simulink model "momentumBasedFlight"  (Simulink 10.3)
settings: Solver=FixedStepAuto  StartTime=0.0  StopTime=Config.simulationTime  FixedStep=Config.tStep  RelTol=1e-3
InitFcn:
  | cd(fileparts(which(bdroot)));
  | initMomentumBasedFlight;
StopFcn:
  | cd(fileparts(which(bdroot)));
  | stopMomentumBasedFlight;
undefined symbols (not defined in the file or in its folder): biasVectorConstraint_feet, Config, confVisualizer, ConstraintMatrix_feet, DiscIntNeverNeededParam, jets_config
undefined symbols (not defined in the file): Frames
libraries: WBToolboxLibrary x25, momentum_flight_control_sublib x2, thrust_estimation_sublib x1, jets_control x1, iDynVisualizer x1
(part 2 of 3)

== system momentumBasedFlight/FLIGHT CONTROLLER (CORE) V2.5 - AERO/Get System State/Change Contact Forces Representation ==
  jointPos : Inport
  w_H_b : Inport  Port=2
  contactForces_WBD : Inport  Port=3
  Change Contact Forces Representation : MATLAB Function  TreatAsAtomicUnit=on
  "CoM6D ->  CoMXYZ1" : Selector  NumberOfDimensions=2  InputPortWidth=7  IndexOptions=Index vector (dialog),Index vector (dialog)  Indices=[1 2 3],[1 2 3]  OutputSizes=1,1
  "CoM6D ->  CoMXYZ3" : Selector  NumberOfDimensions=2  InputPortWidth=7  IndexOptions=Index vector (dialog),Index vector (dialog)  Indices=[1 2 3],[1 2 3]  OutputSizes=1,1
  LFoot Pose : WBToolboxLibrary/Model/Kinematics/ForwardKinematics  frameName=Frames.LFOOT_FRAME
      settings: SourceProductName=WholeBodyToolbox
  Mux : Mux  Inputs=2
  RFoot Pose : WBToolboxLibrary/Model/Kinematics/ForwardKinematics  frameName=Frames.RFOOT_FRAME
      settings: SourceProductName=WholeBodyToolbox
  contactForces : Outport  VectorParamsAs1DForOutWhenUnconnected=off
  tag scope: wrench_LFoot=global, wrench_RFoot=global
  wires:
  contactForces_WBD/1 -> Change Contact Forces Representation/1(contactForces_WBD)
  RFoot Pose/1 -> "CoM6D ->  CoMXYZ3"/1
  "CoM6D ->  CoMXYZ3"/1 -> Change Contact Forces Representation/3(w_R_r_sole)
  LFoot Pose/1 -> "CoM6D ->  CoMXYZ1"/1
  "CoM6D ->  CoMXYZ1"/1 -> Change Contact Forces Representation/2(w_R_l_sole)
  w_H_b/1 -> LFoot Pose/1, RFoot Pose/1
  jointPos/1 -> LFoot Pose/2, RFoot Pose/2
  Change Contact Forces Representation/1(mixed_f_l_sole) -> [wrench_LFoot], Mux/1
  Change Contact Forces Representation/2(mixed_f_r_sole) -> [wrench_RFoot], Mux/2
  Mux/1 -> contactForces/1

== system momentumBasedFlight/Visualizer/Task and Base Frame Kinematics/Combine Rotations ==
  roll : Inport
  pitch : Inport  Port=2
  yaw : Inport  Port=3
  roll_des : Inport  Port=4
  pitch_des : Inport  Port=5
  yaw_des : Inport  Port=6
  Mux : Mux  Inputs=2
  Mux1 : Mux  Inputs=2
  Mux2 : Mux  Inputs=2
  Task rotation combined : Scope  NumInputPorts=3
  wires:
  yaw_des/1 -> Mux2/2
  pitch_des/1 -> Mux1/2
  pitch/1 -> Mux1/1
  roll/1 -> Mux/1
  yaw/1 -> Mux2/1
  roll_des/1 -> Mux/2
  Mux2/1 -> Task rotation combined/3
  Mux1/1 -> Task rotation combined/2
  Mux/1 -> Task rotation combined/1

== system momentumBasedFlight/FLIGHT CONTROLLER (CORE) V2.5 - AERO/Flight Controller RAL-HUMANOIDS V3.0 - AERODYNAMICS/Joint Torque Control for Flying/Integrate Joints Velocity error ==
  jointVel_err : Inport
  Constant : Constant  Value=zeros(Config.N_DOF,1)
  Discrete-Time Integrator1 : DiscreteIntegrator  InitialConditionSource=external  InitialCondition=zeros(Config.N_DOF,1)  SampleTime=Config.tStep  ICPrevOutput=DiscIntNeverNeededParam  ICPrevScaledInput=DiscIntNeverNeededParam
  jointPos_err : Outport  VectorParamsAs1DForOutWhenUnconnected=off
  tag scope: jointPos_err_integral=global
  wires:
  Constant/1 -> Discrete-Time Integrator1/2
  jointVel_err/1 -> Discrete-Time Integrator1/1
  Discrete-Time Integrator1/1 -> [jointPos_err_integral], jointPos_err/1

== system momentumBasedFlight/FLIGHT CONTROLLER (CORE) V2.5 - AERO/Flight Controller RAL-HUMANOIDS V3.0 - AERODYNAMICS/Joint Torque Control for Flying/QP torqueControl ==
  HessianMatrixQP : Inport
  gVectorQP : Inport  Port=2
  ConstraintMatrix_inequality : Inport  Port=3
  biasVectorConstraint_inequality : Inport  Port=4
  feetContactIsActive : Inport  Port=5
  Constant2 : Constant  Value=Config.sat.jointTorquesSaturation
  NOT : Logic  Operator=NOT  IconShape=distinctive  AllPortsSameDT=off  OutDataTypeStr=boolean
  Process QP Inputs Torque Control : MATLAB Function  TreatAsAtomicUnit=on
  QP torqueControl - balancing : Subsystem  TreatAsAtomicUnit=on
  QP torqueControl - flight : Subsystem  TreatAsAtomicUnit=on
  Select QP torqueControl Output : Subsystem
  jointTorques_star : Outport  VectorParamsAs1DForOutWhenUnconnected=off
  exitFlagQP_torqueControl : Outport  Port=2  VectorParamsAs1DForOutWhenUnconnected=off
  wires:
  Select QP torqueControl Output/1(jointTorques_star) -> jointTorques_star/1
  Select QP torqueControl Output/2(exitFlagQP_torqueControl) -> exitFlagQP_torqueControl/1
  QP torqueControl - flight/1(QPStatus_flight) -> Select QP torqueControl Output/4(QPStatus_flight)
  QP torqueControl - flight/2(QPOutput_flight) -> Select QP torqueControl Output/5(QPOutput_flight)
  QP torqueControl - balancing/2(QPOutput_balancing) -> Select QP torqueControl Output/2(QPOutput_balancing)
  QP torqueControl - balancing/1(QPStatus_balancing) -> Select QP torqueControl Output/1(QPStatus_balancing)
  Process QP Inputs Torque Control/1(H_balancing) -> QP torqueControl - balancing/1(H)
  Process QP Inputs Torque Control/2(g_balancing) -> QP torqueControl - balancing/2(g)
  Process QP Inputs Torque Control/3(ub_balancing) -> QP torqueControl - balancing/3(ub)
  Process QP Inputs Torque Control/4(lb_balancing) -> QP torqueControl - balancing/4(lb)
  Process QP Inputs Torque Control/5(Aeq_balancing) -> QP torqueControl - balancing/5(AEq)
  Process QP Inputs Torque Control/6(lbEq_balancing) -> QP torqueControl - balancing/6(lbEq)
  Process QP Inputs Torque Control/7(ubEq_balancing) -> QP torqueControl - balancing/7(ubEq)
  Process QP Inputs Torque Control/11(lb_flight) -> QP torqueControl - flight/4(lb)
  Process QP Inputs Torque Control/10(ub_flight) -> QP torqueControl - flight/3(ub)
  Process QP Inputs Torque Control/9(g_flight) -> QP torqueControl - flight/2(g)
  Process QP Inputs Torque Control/8(H_flight) -> QP torqueControl - flight/1(H)
  Constant2/1 -> Process QP Inputs Torque Control/5(jointTorquesSaturation)
  gVectorQP/1 -> Process QP Inputs Torque Control/2(gVectorQP)
  HessianMatrixQP/1 -> Process QP Inputs Torque Control/1(HessianMatrixQP)
  ConstraintMatrix_inequality/1 -> Process QP Inputs Torque Control/3(InequalityConstrMatrix)
  biasVectorConstraint_inequality/1 -> Process QP Inputs Torque Control/4(biasVectorInequalityConstr)
  NOT/1 -> QP torqueControl - flight/Enable
  feetContactIsActive/1 -> NOT/1, QP torqueControl - balancing/Enable, Select QP torqueControl Output/3(feetContactIsActive)

== system momentumBasedFlight/FLIGHT CONTROLLER (CORE) V2.5 - AERO/Flight Controller RAL-HUMANOIDS V3.0 - AERODYNAMICS/Joint Torque Control for Flying/Torque Derivative Saturation ==
  jointTorques_star : Inport
  Constant1 : Constant  Value=Config.tStep
  Constant2 : Constant  Value=Config.sat.jointTorquesDotMax
  Saturate Torque Derivative : MATLAB Function  TreatAsAtomicUnit=on
  "holder " : WBToolboxLibrary/Utilities/holder 
      settings: SourceProductName=WholeBodyToolbox
  jointTorques_star_sat : Outport  VectorParamsAs1DForOutWhenUnconnected=off
  wires:
  Constant2/1 -> Saturate Torque Derivative/4(uDotMax)
  Constant1/1 -> Saturate Torque Derivative/3(tStep)
  "holder "/1 -> Saturate Torque Derivative/2(u_0)
  Saturate Torque Derivative/1(uSat) -> jointTorques_star_sat/1
  jointTorques_star/1 -> Saturate Torque Derivative/1(u), "holder "/1

== system momentumBasedFlight/FLIGHT CONTROLLER (CORE) V2.5 - AERO/Flight Controller RAL-HUMANOIDS V3.0 - AERODYNAMICS/Momentum Control for Flying/Jet Control ==
  jetDerivatives_des : Inport
  jetsIntensities : Inport  Port=2
  4Jets_EKF : thrust_estimation_sublib/For Test-bench/4Jets_EKF  Config=Config
      settings: SourceProductName=iRonCub Library
  Feedback linearization 4-jets control : jets_control/Feedback linearization 4-jets control  Conf=Config
      settings: SourceProductName=iRonCub Library
  throttle : Outport
  wires:
  4Jets_EKF/1 -> Feedback linearization 4-jets control/1
  Feedback linearization 4-jets control/1 -> throttle/1, 4Jets_EKF/1
  jetsIntensities/1 -> 4Jets_EKF/2
  jetDerivatives_des/1 -> Feedback linearization 4-jets control/2

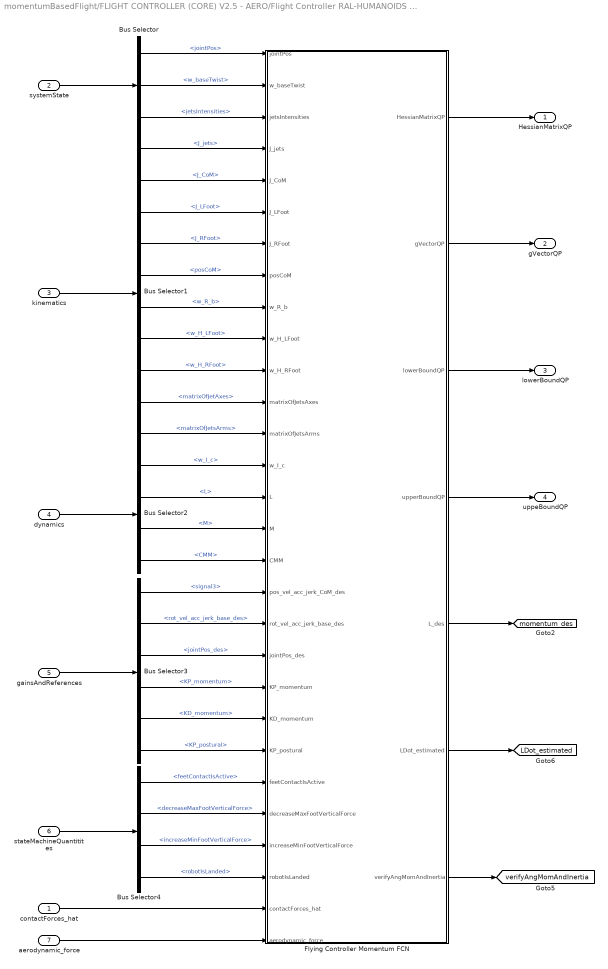
== system momentumBasedFlight/FLIGHT CONTROLLER (CORE) V2.5 - AERO/Flight Controller RAL-HUMANOIDS V3.0 - AERODYNAMICS/Momentum Control for Flying/Momentum Control ==
  contactForces_hat : Inport
  systemState : Inport  Port=2
  kinematics : Inport  Port=3
  dynamics : Inport  Port=4
  gainsAndReferences : Inport  Port=5
  stateMachineQuantitites : Inport  Port=6
  aerodynamic_force : Inport  Port=7
  Bus Selector : BusSelector  OutputSignals=jointPos,w_baseTwist,jetsIntensities
  Bus Selector1 : BusSelector  OutputSignals=J_jets,J_CoM,J_LFoot,J_RFoot,posCoM,w_R_b,w_H_LFoot,w_H_RFoot,matrixOfJetAxes,matrixOfJetsArms
  Bus Selector2 : BusSelector  OutputSignals=w_I_c,L,M,CMM
  Bus Selector3 : BusSelector  OutputSignals=signal3,rot_vel_acc_jerk_base_des,jointPos_des,KP_momentum,KD_momentum,KP_postural
  Bus Selector4 : BusSelector  OutputSignals=feetContactIsActive,decreaseMaxFootVerticalForce,increaseMinFootVerticalForce,robotIsLanded
  "Flying Controller Momentum FCN " : MATLAB Function  TreatAsAtomicUnit=on
  HessianMatrixQP : Outport  VectorParamsAs1DForOutWhenUnconnected=off
  gVectorQP : Outport  Port=2  VectorParamsAs1DForOutWhenUnconnected=off
  lowerBoundQP : Outport  Port=3  VectorParamsAs1DForOutWhenUnconnected=off
  uppeBoundQP : Outport  Port=4  VectorParamsAs1DForOutWhenUnconnected=off
  tag scope: LDot_estimated=global, momentum_des=global, verifyAngMomAndInertia=global
  wires:
  contactForces_hat/1 -> "Flying Controller Momentum FCN "/28(contactForces_hat)
  Bus Selector4/4 -> "Flying Controller Momentum FCN "/27(robotIsLanded)  "<robotIsLanded>"
  Bus Selector4/3 -> "Flying Controller Momentum FCN "/26(increaseMinFootVerticalForce)  "<increaseMinFootVerticalForce>"
  Bus Selector4/2 -> "Flying Controller Momentum FCN "/25(decreaseMaxFootVerticalForce)  "<decreaseMaxFootVerticalForce>"
  Bus Selector2/1 -> "Flying Controller Momentum FCN "/14(w_I_c)  "<w_I_c>"
  Bus Selector1/10 -> "Flying Controller Momentum FCN "/13(matrixOfJetsArms)  "<matrixOfJetsArms>"
  Bus Selector1/9 -> "Flying Controller Momentum FCN "/12(matrixOfJetsAxes)  "<matrixOfJetAxes>"
  Bus Selector3/1 -> "Flying Controller Momentum FCN "/18(pos_vel_acc_jerk_CoM_des)  "<signal3>"
  Bus Selector1/6 -> "Flying Controller Momentum FCN "/9(w_R_b)  "<w_R_b>"
  Bus Selector3/2 -> "Flying Controller Momentum FCN "/19(rot_vel_acc_jerk_base_des)  "<rot_vel_acc_jerk_base_des>"
  Bus Selector1/5 -> "Flying Controller Momentum FCN "/8(posCoM)  "<posCoM>"
  "Flying Controller Momentum FCN "/5(L_des) -> [momentum_des]
  Bus Selector3/6 -> "Flying Controller Momentum FCN "/23(KP_postural)  "<KP_postural>"
  Bus Selector2/2 -> "Flying Controller Momentum FCN "/15(L)  "<L>"
  Bus Selector1/7 -> "Flying Controller Momentum FCN "/10(w_H_LFoot)  "<w_H_LFoot>"
  Bus Selector3/5 -> "Flying Controller Momentum FCN "/22(KD_momentum)  "<KD_momentum>"
  "Flying Controller Momentum FCN "/6(LDot_estimated) -> [LDot_estimated]
  Bus Selector2/3 -> "Flying Controller Momentum FCN "/16(M)  "<M>"
  Bus Selector2/4 -> "Flying Controller Momentum FCN "/17(CMM)  "<CMM>"
  Bus Selector1/8 -> "Flying Controller Momentum FCN "/11(w_H_RFoot)  "<w_H_RFoot>"
  Bus Selector1/4 -> "Flying Controller Momentum FCN "/7(J_RFoot)  "<J_RFoot>"
  Bus Selector/3 -> "Flying Controller Momentum FCN "/3(jetsIntensities)  "<jetsIntensities>"
  gainsAndReferences/1 -> Bus Selector3/1
  Bus Selector1/2 -> "Flying Controller Momentum FCN "/5(J_CoM)  "<J_CoM>"
  dynamics/1 -> Bus Selector2/1
  Bus Selector3/4 -> "Flying Controller Momentum FCN "/21(KP_momentum)  "<KP_momentum>"
  "Flying Controller Momentum FCN "/3(lowerBoundQP) -> lowerBoundQP/1
  stateMachineQuantitites/1 -> Bus Selector4/1
  "Flying Controller Momentum FCN "/7(verifyAngMomAndInertia) -> [verifyAngMomAndInertia]
  Bus Selector4/1 -> "Flying Controller Momentum FCN "/24(feetContactIsActive)  "<feetContactIsActive>"
  "Flying Controller Momentum FCN "/2(gVectorQP) -> gVectorQP/1
  "Flying Controller Momentum FCN "/4(upperBoundQP) -> uppeBoundQP/1
  "Flying Controller Momentum FCN "/1(HessianMatrixQP) -> HessianMatrixQP/1
  Bus Selector/2 -> "Flying Controller Momentum FCN "/2(w_baseTwist)  "<w_baseTwist>"
  Bus Selector1/1 -> "Flying Controller Momentum FCN "/4(J_jets)  "<J_jets>"
  Bus Selector/1 -> "Flying Controller Momentum FCN "/1(jointPos)  "<jointPos>"
  kinematics/1 -> Bus Selector1/1
  Bus Selector1/3 -> "Flying Controller Momentum FCN "/6(J_LFoot)  "<J_LFoot>"
  Bus Selector3/3 -> "Flying Controller Momentum FCN "/20(jointPos_des)  "<jointPos_des>"
  systemState/1 -> Bus Selector/1
  aerodynamic_force/1 -> "Flying Controller Momentum FCN "/29(aerodynamic_force)

== system momentumBasedFlight/FLIGHT CONTROLLER (CORE) V2.5 - AERO/Flight Controller RAL-HUMANOIDS V3.0 - AERODYNAMICS/Momentum Control for Flying/QP Solver and Integrate Contact Forces Derivative ==
  HessianMatrixQP : Inport
  gVectorQP : Inport  Port=2
  lowerBoundQP : Inport  Port=3
  upperBoundQP : Inport  Port=4
  stateMachineQuantities : Inport  Port=5
  systemState : Inport  Port=6
  Bus Selector1 : BusSelector  OutputSignals=feetContactIsActive
  Bus Selector2 : BusSelector  OutputSignals=contactForces
  Integrate the Contact Forces Derivative : Subsystem
  QP momentumControl : Subsystem
  contactForces_star : Outport  VectorParamsAs1DForOutWhenUnconnected=off
  jetsIntensitiesDot_star : Outport  Port=2  VectorParamsAs1DForOutWhenUnconnected=off
  jointVel_star : Outport  Port=3  VectorParamsAs1DForOutWhenUnconnected=off
  tag scope: contactForces_star=global, exitFlagQP_momentumControl=global, jetsIntensitiesDot_star=global, jointVel_star=global
  wires:
  systemState/1 -> Bus Selector2/1
  Bus Selector2/1 -> Integrate the Contact Forces Derivative/2(contactForces)  "<contactForces>"
  Bus Selector1/1 -> Integrate the Contact Forces Derivative/3(feetContactIsActive), QP momentumControl/5(feetContactIsActive)  "<feetContactIsActive>"
  QP momentumControl/3(jointVel_star) -> jointVel_star/1, [jointVel_star]
  QP momentumControl/1(jetsIntensitiesDot_star) -> [jetsIntensitiesDot_star], jetsIntensitiesDot_star/1
  HessianMatrixQP/1 -> QP momentumControl/1(HessianMatrixQP)
  stateMachineQuantities/1 -> Bus Selector1/1
  gVectorQP/1 -> QP momentumControl/2(gVectorQP)
  QP momentumControl/4(exitFlagQP_momentumControl) -> [exitFlagQP_momentumControl]
  upperBoundQP/1 -> QP momentumControl/4(upperBoundQP)
  lowerBoundQP/1 -> QP momentumControl/3(lowerBoundQP)
  QP momentumControl/2(contactForcesDot_star) -> Integrate the Contact Forces Derivative/1(contactForcesDot_star)
  Integrate the Contact Forces Derivative/1(contactForces_star) -> contactForces_star/1, [contactForces_star]

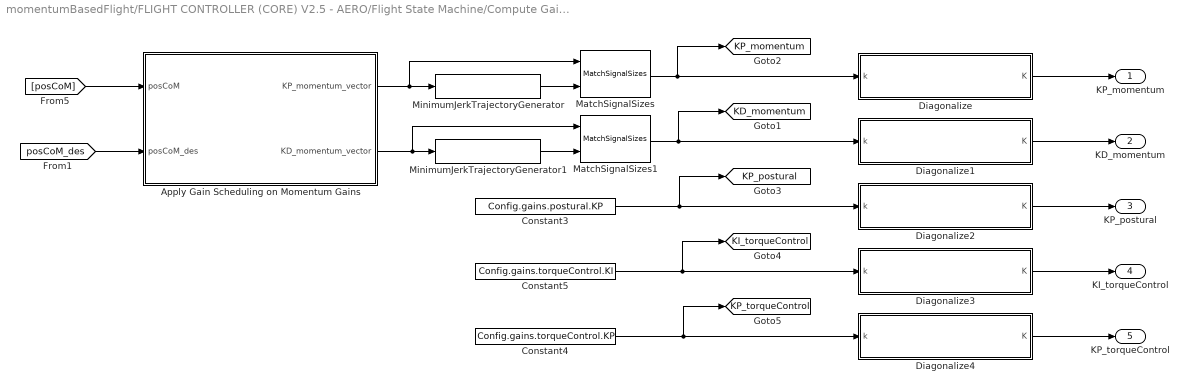
== system momentumBasedFlight/FLIGHT CONTROLLER (CORE) V2.5 - AERO/Flight State Machine/Compute Gains And References/Compute Gains ==
  Apply Gain Scheduling on Momentum Gains : MATLAB Function  TreatAsAtomicUnit=on
  Constant3 : Constant  Value=Config.gains.postural.KP
  Constant4 : Constant  Value=Config.gains.torqueControl.KP
  Constant5 : Constant  Value=Config.gains.torqueControl.KI
  Diagonalize : MATLAB Function  TreatAsAtomicUnit=on
  Diagonalize1 : MATLAB Function  TreatAsAtomicUnit=on
  Diagonalize2 : MATLAB Function  TreatAsAtomicUnit=on
  Diagonalize3 : MATLAB Function  TreatAsAtomicUnit=on
  Diagonalize4 : MATLAB Function  TreatAsAtomicUnit=on
  MatchSignalSizes : WBToolboxLibrary/Utilities/MatchSignalSizes
      settings: SourceProductName=WholeBodyToolbox
  MatchSignalSizes1 : WBToolboxLibrary/Utilities/MatchSignalSizes
      settings: SourceProductName=WholeBodyToolbox
  MinimumJerkTrajectoryGenerator : WBToolboxLibrary/Utilities/MinimumJerkTrajectoryGenerator  externalSettlingTime=off  settlingTime=Config.settlingTime_gainScheduling  sampleTime=Config.tStep  resetOnSettlingTime=off  firstDerivatives=off  secondDerivatives=off  explicitInitialValue=off
      settings: SourceProductName=WholeBodyToolbox
  MinimumJerkTrajectoryGenerator1 : WBToolboxLibrary/Utilities/MinimumJerkTrajectoryGenerator  externalSettlingTime=off  settlingTime=Config.settlingTime_gainScheduling  sampleTime=Config.tStep  resetOnSettlingTime=off  firstDerivatives=off  secondDerivatives=off  explicitInitialValue=off
      settings: SourceProductName=WholeBodyToolbox
  KP_momentum : Outport  VectorParamsAs1DForOutWhenUnconnected=off
  KD_momentum : Outport  Port=2  VectorParamsAs1DForOutWhenUnconnected=off
  KP_postural : Outport  Port=3  VectorParamsAs1DForOutWhenUnconnected=off
  KI_torqueControl : Outport  Port=4  VectorParamsAs1DForOutWhenUnconnected=off
  KP_torqueControl : Outport  Port=5  VectorParamsAs1DForOutWhenUnconnected=off
  tag scope: KD_momentum=global, KI_torqueControl=global, KP_momentum=global, KP_postural=global, KP_torqueControl=global
  wires:
  Constant4/1 -> Diagonalize4/1(k), [KP_torqueControl]
  Constant5/1 -> Diagonalize3/1(k), [KI_torqueControl]
  Constant3/1 -> Diagonalize2/1(k), [KP_postural]
  MatchSignalSizes1/1 -> Diagonalize1/1(k), [KD_momentum]
  MatchSignalSizes/1 -> [KP_momentum], Diagonalize/1(k)
  Diagonalize4/1(K) -> KP_torqueControl/1
  Diagonalize3/1(K) -> KI_torqueControl/1
  Diagonalize2/1(K) -> KP_postural/1
  Diagonalize1/1(K) -> KD_momentum/1
  Diagonalize/1(K) -> KP_momentum/1
  [posCoM] -> Apply Gain Scheduling on Momentum Gains/1(posCoM)
  [posCoM_des] -> Apply Gain Scheduling on Momentum Gains/2(posCoM_des)
  Apply Gain Scheduling on Momentum Gains/1(KP_momentum_vector) -> MatchSignalSizes/1, MinimumJerkTrajectoryGenerator/1
  Apply Gain Scheduling on Momentum Gains/2(KD_momentum_vector) -> MatchSignalSizes1/1, MinimumJerkTrajectoryGenerator1/1
  MinimumJerkTrajectoryGenerator/1 -> MatchSignalSizes/2
  MinimumJerkTrajectoryGenerator1/1 -> MatchSignalSizes1/2

== system momentumBasedFlight/FLIGHT CONTROLLER (CORE) V2.5 - AERO/Flight State Machine/Compute Gains And References/High-speed Flight Trajectory Generator ==
  posCoM_init : Inport
  Clock1 : Clock
  "Trajectory Design for High Speed Motion " : MATLAB Function  TreatAsAtomicUnit=on
  pos_vel_acc_jerk_CoM_des_high_speed : Outport
  turbo_mode_hs : Outport  Port=2
  wires:
  posCoM_init/1 -> "Trajectory Design for High Speed Motion "/2(posCoM_init)
  "Trajectory Design for High Speed Motion "/1(pos_vel_acc_jerk_CoM_des) -> pos_vel_acc_jerk_CoM_des_high_speed/1
  Clock1/1 -> "Trajectory Design for High Speed Motion "/1(t)
  "Trajectory Design for High Speed Motion "/2(turbo_mode_hs) -> turbo_mode_hs/1

== system momentumBasedFlight/FLIGHT CONTROLLER (CORE) V2.5 - AERO/Flight State Machine/Compute Gains And References/Select Planned Trajectory ==
  pos_vel_acc_jerk_CoM_des_ls : Inport
  use_high_speed_traj : Inport  Port=2
  pos_vel_acc_jerk_CoM_des_hs : Inport  Port=3
  Select Trajectory : Switch  Criteria=u2 > Threshold
  pos_vel_acc_jerk_CoM_des : Outport
  wires:
  Select Trajectory/1 -> pos_vel_acc_jerk_CoM_des/1
  use_high_speed_traj/1 -> Select Trajectory/2
  pos_vel_acc_jerk_CoM_des_hs/1 -> Select Trajectory/1
  pos_vel_acc_jerk_CoM_des_ls/1 -> Select Trajectory/3

== system momentumBasedFlight/FLIGHT CONTROLLER (CORE) V2.5 - AERO/Flight State Machine/Compute Gains And References/Smooth CoM and Base References ==
  pos_vel_acc_jerk_CoM_des : Inport
  smoothingTimeCoMPos : Inport  Port=2
  gainSmoothingBaseRot : Inport  Port=3
  rot_vel_acc_jerk_base_des : Inport  Port=4
  Constant : Constant  Value=Config.references.SMOOTH_BASE_ROT_REFERENCES
  Constant1 : Constant  Value=Config.references.SMOOTH_COM_POS_REFERENCES
  Smooth Position References : Subsystem
  Smooth Reference Orientations : Subsystem
  Switch : Switch  Criteria=u2 > Threshold
  Switch2 : Switch  Criteria=u2 > Threshold
  pos_vel_acc_jerk_CoM_des_smooth : Outport  VectorParamsAs1DForOutWhenUnconnected=off
  rot_vel_acc_jerk_base_des_smooth : Outport  Port=2  VectorParamsAs1DForOutWhenUnconnected=off
  wires:
  Constant/1 -> Switch2/2
  Smooth Reference Orientations/1(rot_acc_vel_jerk_base_des_smooth) -> Switch2/1
  gainSmoothingBaseRot/1 -> Smooth Reference Orientations/2(gainSmoothingBaseRot), Switch2/3
  rot_vel_acc_jerk_base_des/1 -> Smooth Reference Orientations/1(rot_vel_acc_jerk_base_des)
  Constant1/1 -> Switch/2
  Switch/1 -> pos_vel_acc_jerk_CoM_des_smooth/1
  Switch2/1 -> rot_vel_acc_jerk_base_des_smooth/1
  pos_vel_acc_jerk_CoM_des/1 -> Smooth Position References/2(pos_vel_acc_jerk_CoM_des), Switch/3
  smoothingTimeCoMPos/1 -> Smooth Position References/1(smoothingTimeCoMPos)
  Smooth Position References/1(pos_vel_acc_jerk_CoM_des_smooth) -> Switch/1

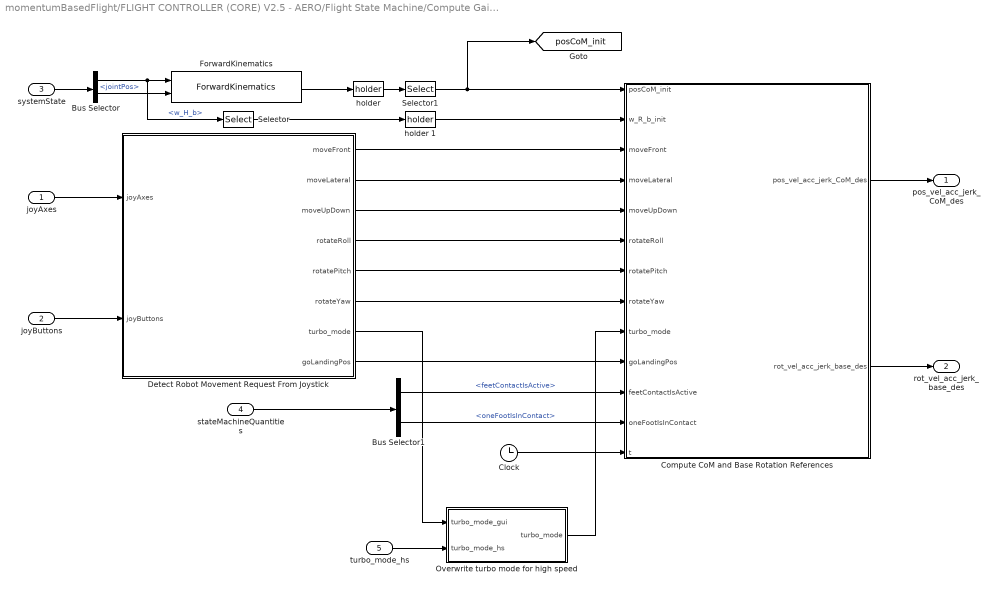
== system momentumBasedFlight/FLIGHT CONTROLLER (CORE) V2.5 - AERO/Flight State Machine/Compute Gains And References/Trajectory Generator ==
  joyAxes : Inport
  joyButtons : Inport  Port=2
  systemState : Inport  Port=3
  stateMachineQuantities : Inport  Port=4
  turbo_mode_hs : Inport  Port=5
  Bus Selector : BusSelector  OutputSignals=w_H_b,jointPos
  Bus Selector1 : BusSelector  OutputSignals=feetContactIsActive,oneFootIsInContact
  Clock : Clock
  Compute CoM and Base Rotation References : MATLAB Function  TreatAsAtomicUnit=on
  Detect Robot Movement Request From Joystick : MATLAB Function  TreatAsAtomicUnit=on
  ForwardKinematics : WBToolboxLibrary/Model/Kinematics/ForwardKinematics  frameName=Frames.COM_FRAME
      settings: SourceProductName=WholeBodyToolbox
  Overwrite turbo mode for high speed : Subsystem
  Selector : Selector  NumberOfDimensions=2  InputPortWidth=3  IndexOptions=Index vector (dialog),Index vector (dialog)  Indices=[1 2 3],[1 2 3]  OutputSizes=1,1
  Selector1 : Selector  NumberOfDimensions=2  InputPortWidth=3  IndexOptions=Index vector (dialog),Index vector (dialog)  Indices=[1 2 3],[4]  OutputSizes=1,1
  "holder " : WBToolboxLibrary/Utilities/holder 
      settings: SourceProductName=WholeBodyToolbox
  holder 1 : WBToolboxLibrary/Utilities/holder 
      settings: SourceProductName=WholeBodyToolbox
  pos_vel_acc_jerk_CoM_des : Outport  VectorParamsAs1DForOutWhenUnconnected=off
  rot_vel_acc_jerk_base_des : Outport  Port=2  VectorParamsAs1DForOutWhenUnconnected=off
  tag scope: posCoM_init=global
  wires:
  Detect Robot Movement Request From Joystick/7(turbo_mode) -> Overwrite turbo mode for high speed/1(turbo_mode_gui)
  Detect Robot Movement Request From Joystick/1(moveFront) -> Compute CoM and Base Rotation References/3(moveFront)
  "holder "/1 -> Selector1/1
  Bus Selector/2 -> ForwardKinematics/2  "<jointPos>"
  Detect Robot Movement Request From Joystick/3(moveUpDown) -> Compute CoM and Base Rotation References/5(moveUpDown)
  Detect Robot Movement Request From Joystick/2(moveLateral) -> Compute CoM and Base Rotation References/4(moveLateral)
  stateMachineQuantities/1 -> Bus Selector1/1
  Detect Robot Movement Request From Joystick/5(rotatePitch) -> Compute CoM and Base Rotation References/7(rotatePitch)
  Bus Selector1/1 -> Compute CoM and Base Rotation References/11(feetContactIsActive)  "<feetContactIsActive>"
  Selector/1 -> holder 1/1
  Bus Selector/1 -> ForwardKinematics/1, Selector/1  "<w_H_b>"
  holder 1/1 -> Compute CoM and Base Rotation References/2(w_R_b_init)
  ForwardKinematics/1 -> "holder "/1
  Detect Robot Movement Request From Joystick/4(rotateRoll) -> Compute CoM and Base Rotation References/6(rotateRoll)
  Compute CoM and Base Rotation References/1(pos_vel_acc_jerk_CoM_des) -> pos_vel_acc_jerk_CoM_des/1
  Detect Robot Movement Request From Joystick/6(rotateYaw) -> Compute CoM and Base Rotation References/8(rotateYaw)
  Clock/1 -> Compute CoM and Base Rotation References/13(t)
  systemState/1 -> Bus Selector/1
  joyAxes/1 -> Detect Robot Movement Request From Joystick/1(joyAxes)
  joyButtons/1 -> Detect Robot Movement Request From Joystick/2(joyButtons)
  Compute CoM and Base Rotation References/2(rot_vel_acc_jerk_base_des) -> rot_vel_acc_jerk_base_des/1
  Selector1/1 -> [posCoM_init], Compute CoM and Base Rotation References/1(posCoM_init)
  Detect Robot Movement Request From Joystick/8(goLandingPos) -> Compute CoM and Base Rotation References/10(goLandingPos)
  Bus Selector1/2 -> Compute CoM and Base Rotation References/12(oneFootIsInContact)  "<oneFootIsInContact>"
  turbo_mode_hs/1 -> Overwrite turbo mode for high speed/2(turbo_mode_hs)
  Overwrite turbo mode for high speed/1(turbo_mode) -> Compute CoM and Base Rotation References/9(turbo_mode)

== system momentumBasedFlight/FLIGHT CONTROLLER (CORE) V2.5 - AERO/Flight Controller RAL-HUMANOIDS V3.0 - AERODYNAMICS/Joint Torque Control for Flying/QP torqueControl/QP torqueControl - balancing ==
  H : Inport
  g : Inport  Port=2
  ub : Inport  Port=3
  lb : Inport  Port=4
  AEq : Inport  Port=5
  lbEq : Inport  Port=6
  ubEq : Inport  Port=7
  Enable : EnablePort
  Combine Bounds and Inequalities : MATLAB Function  TreatAsAtomicUnit=on
  MatchSignalSizes : WBToolboxLibrary/Utilities/MatchSignalSizes
      settings: SourceProductName=WholeBodyToolbox
  QP : WBToolboxLibrary/Utilities/QP  lbA=on  ubA=on  lb=off  ub=off  computeObjVal=off  stopIfFails=off
      settings: SourceProductName=WholeBodyToolbox
  QPStatus_balancing : Outport  VectorParamsAs1DForOutWhenUnconnected=off
  QPOutput_balancing : Outport  Port=2  VectorParamsAs1DForOutWhenUnconnected=off
  wires:
  Combine Bounds and Inequalities/3(ubEq_combined) -> QP/5
  Combine Bounds and Inequalities/2(lbEq_combined) -> QP/4
  Combine Bounds and Inequalities/1(AEq_combined) -> QP/3
  ub/1 -> Combine Bounds and Inequalities/5(ub)
  lb/1 -> Combine Bounds and Inequalities/4(lb)
  ubEq/1 -> Combine Bounds and Inequalities/3(ubEq)
  lbEq/1 -> Combine Bounds and Inequalities/2(lbEq)
  AEq/1 -> Combine Bounds and Inequalities/1(AEq)
  g/1 -> QP/2, MatchSignalSizes/1
  H/1 -> QP/1
  QP/1 -> MatchSignalSizes/2
  MatchSignalSizes/1 -> QPOutput_balancing/1
  QP/2 -> QPStatus_balancing/1

== system momentumBasedFlight/FLIGHT CONTROLLER (CORE) V2.5 - AERO/Flight Controller RAL-HUMANOIDS V3.0 - AERODYNAMICS/Joint Torque Control for Flying/QP torqueControl/QP torqueControl - flight ==
  H : Inport
  g : Inport  Port=2
  ub : Inport  Port=3
  lb : Inport  Port=4
  Enable : EnablePort
  MatchSignalSizes : WBToolboxLibrary/Utilities/MatchSignalSizes
      settings: SourceProductName=WholeBodyToolbox
  QP : WBToolboxLibrary/Utilities/QP  lbA=off  ubA=off  lb=on  ub=on  computeObjVal=off  stopIfFails=off
      settings: SourceProductName=WholeBodyToolbox
  QPStatus_flight : Outport  VectorParamsAs1DForOutWhenUnconnected=off
  QPOutput_flight : Outport  Port=2  VectorParamsAs1DForOutWhenUnconnected=off
  wires:
  ub/1 -> QP/4
  g/1 -> QP/2, MatchSignalSizes/1
  H/1 -> QP/1
  QP/1 -> MatchSignalSizes/2
  MatchSignalSizes/1 -> QPOutput_flight/1
  lb/1 -> QP/3
  QP/2 -> QPStatus_flight/1

== system momentumBasedFlight/FLIGHT CONTROLLER (CORE) V2.5 - AERO/Flight Controller RAL-HUMANOIDS V3.0 - AERODYNAMICS/Joint Torque Control for Flying/QP torqueControl/Select QP torqueControl Output ==
  QPStatus_balancing : Inport
  QPOutput_balancing : Inport  Port=2
  feetContactIsActive : Inport  Port=3
  QPStatus_flight : Inport  Port=4
  QPOutput_flight : Inport  Port=5
  Demux : Demux  Outputs=[12;Config.N_DOF]
  Switch : Switch  Criteria=u2 > Threshold
  Switch1 : Switch  Criteria=u2 > Threshold
  contactForces_QP : Terminator
  jointTorques_star : Outport  VectorParamsAs1DForOutWhenUnconnected=off
  exitFlagQP_torqueControl : Outport  Port=2  VectorParamsAs1DForOutWhenUnconnected=off
  wires:
  Demux/2 -> Switch1/1
  Demux/1 -> contactForces_QP/1
  QPOutput_flight/1 -> Switch1/3
  QPOutput_balancing/1 -> Demux/1
  Switch/1 -> exitFlagQP_torqueControl/1
  QPStatus_flight/1 -> Switch/3
  QPStatus_balancing/1 -> Switch/1
  feetContactIsActive/1 -> Switch/2, Switch1/2
  Switch1/1 -> jointTorques_star/1

== system momentumBasedFlight/FLIGHT CONTROLLER (CORE) V2.5 - AERO/Flight Controller RAL-HUMANOIDS V3.0 - AERODYNAMICS/Momentum Control for Flying/QP Solver and Integrate Contact Forces Derivative/Integrate the Contact Forces Derivative ==
  contactForcesDot_star : Inport
  contactForces : Inport  Port=2
  feetContactIsActive : Inport  Port=3
  Discrete-Time Integrator1 : DiscreteIntegrator  ExternalReset=either  InitialConditionSource=external  InitialCondition=zeros(6,1)  SampleTime=Config.tStep  ICPrevOutput=DiscIntNeverNeededParam  ICPrevScaledInput=DiscIntNeverNeededParam
  Select Integrator Initial Condition : MATLAB Function  TreatAsAtomicUnit=on
  deadZone : Subsystem
  contactForces_star : Outport  VectorParamsAs1DForOutWhenUnconnected=off
  tag scope: contactForcesDot_star=global
  wires:
  Select Integrator Initial Condition/1(contactForces_0) -> Discrete-Time Integrator1/3
  feetContactIsActive/1 -> Discrete-Time Integrator1/2, Select Integrator Initial Condition/1(feetContactIsActive)
  contactForces/1 -> Select Integrator Initial Condition/2(contactForces)
  deadZone/1(u_cut) -> Discrete-Time Integrator1/1
  contactForcesDot_star/1 -> [contactForcesDot_star], deadZone/1(u)
  Discrete-Time Integrator1/1 -> contactForces_star/1

== system momentumBasedFlight/FLIGHT CONTROLLER (CORE) V2.5 - AERO/Flight Controller RAL-HUMANOIDS V3.0 - AERODYNAMICS/Momentum Control for Flying/QP Solver and Integrate Contact Forces Derivative/QP momentumControl ==
  HessianMatrixQP : Inport
  gVectorQP : Inport  Port=2
  lowerBoundQP : Inport  Port=3
  upperBoundQP : Inport  Port=4
  feetContactIsActive : Inport  Port=5
  NOT : Logic  Operator=NOT  IconShape=distinctive  AllPortsSameDT=off  OutDataTypeStr=boolean
  Process QP Inputs Momentum Control : MATLAB Function  TreatAsAtomicUnit=on
  QP momentumControl - balancing : Subsystem  TreatAsAtomicUnit=on
  QP momentumControl - flight : Subsystem  TreatAsAtomicUnit=on
  Select QP momentumControl Output : Subsystem
  jetsIntensitiesDot_star : Outport  VectorParamsAs1DForOutWhenUnconnected=off
  contactForcesDot_star : Outport  Port=2  VectorParamsAs1DForOutWhenUnconnected=off
  jointVel_star : Outport  Port=3  VectorParamsAs1DForOutWhenUnconnected=off
  exitFlagQP_momentumControl : Outport  Port=4  VectorParamsAs1DForOutWhenUnconnected=off
  wires:
  QP momentumControl - flight/2(QPOutput_flight) -> Select QP momentumControl Output/5(QPOutput_flight)
  QP momentumControl - flight/1(QPStatus_flight) -> Select QP momentumControl Output/4(QPStatus_flight)
  QP momentumControl - balancing/2(QPOutput_balancing) -> Select QP momentumControl Output/2(QPOutput_balancing)
  QP momentumControl - balancing/1(QPStatus_balancing) -> Select QP momentumControl Output/1(QPStatus_balancing)
  Select QP momentumControl Output/4(exitFlagQP_momentumControl) -> exitFlagQP_momentumControl/1
  NOT/1 -> QP momentumControl - flight/Enable
  Process QP Inputs Momentum Control/8(lb_flight) -> QP momentumControl - flight/4(lb)
  Process QP Inputs Momentum Control/7(ub_flight) -> QP momentumControl - flight/3(ub)
  Process QP Inputs Momentum Control/4(lb_balancing) -> QP momentumControl - balancing/4(lb)
  Process QP Inputs Momentum Control/3(ub_balancing) -> QP momentumControl - balancing/3(ub)
  Process QP Inputs Momentum Control/6(g_flight) -> QP momentumControl - flight/2(g)
  Process QP Inputs Momentum Control/5(H_flight) -> QP momentumControl - flight/1(H)
  Process QP Inputs Momentum Control/2(g_balancing) -> QP momentumControl - balancing/2(g)
  Process QP Inputs Momentum Control/1(H_balancing) -> QP momentumControl - balancing/1(H)
  Select QP momentumControl Output/2(contactForcesDot_star) -> contactForcesDot_star/1
  Select QP momentumControl Output/3(jointVel_star) -> jointVel_star/1
  Select QP momentumControl Output/1(jetsIntensitiesDot_star) -> jetsIntensitiesDot_star/1
  HessianMatrixQP/1 -> Process QP Inputs Momentum Control/1(HessianMatrixQP)
  upperBoundQP/1 -> Process QP Inputs Momentum Control/4(upperBoundQP)
  feetContactIsActive/1 -> QP momentumControl - balancing/Enable, NOT/1, Select QP momentumControl Output/3(feetContactIsActive)
  lowerBoundQP/1 -> Process QP Inputs Momentum Control/3(lowerBoundQP)
  gVectorQP/1 -> Process QP Inputs Momentum Control/2(gVectorQP)

== system momentumBasedFlight/FLIGHT CONTROLLER (CORE) V2.5 - AERO/Flight State Machine/Compute Gains And References/Smooth CoM and Base References/Smooth Position References ==
  smoothingTimeCoMPos : Inport
  pos_vel_acc_jerk_CoM_des : Inport  Port=2
  "CoM6D ->  CoMXYZ5" : Selector  NumberOfDimensions=2  InputPortWidth=7  IndexOptions=Index vector (dialog),Index vector (dialog)  Indices=[1 2 3],[1]  OutputSizes=1,1
  Compute Smooth Jerk Reference : WBToolboxLibrary/Utilities/MinimumJerkTrajectoryGenerator  externalSettlingTime=off  settlingTime=Config.references.com.tSmoothingCoMAcc  sampleTime=Config.tStep  resetOnSettlingTime=off  firstDerivatives=on  secondDerivatives=off  explicitInitialValue=off
      settings: SourceProductName=WholeBodyToolbox
  Matrix Concatenate : Concatenate  NumInputs=4  Mode=Multidimensional array  ConcatenateDimension=2
  MinimumJerkTrajectoryGenerator : WBToolboxLibrary/Utilities/MinimumJerkTrajectoryGenerator  externalSettlingTime=on  settlingTime=3  sampleTime=Config.tStep  resetOnSettlingTime=off  firstDerivatives=on  secondDerivatives=on  explicitInitialValue=off
      settings: SourceProductName=WholeBodyToolbox
  Terminator : Terminator
  pos_vel_acc_jerk_CoM_des_smooth : Outport  VectorParamsAs1DForOutWhenUnconnected=off
  wires:
  Compute Smooth Jerk Reference/2 -> Matrix Concatenate/4
  Compute Smooth Jerk Reference/1 -> Terminator/1
  MinimumJerkTrajectoryGenerator/3 -> Compute Smooth Jerk Reference/1, Matrix Concatenate/3
  MinimumJerkTrajectoryGenerator/2 -> Matrix Concatenate/2
  "CoM6D ->  CoMXYZ5"/1 -> MinimumJerkTrajectoryGenerator/1
  Matrix Concatenate/1 -> pos_vel_acc_jerk_CoM_des_smooth/1
  MinimumJerkTrajectoryGenerator/1 -> Matrix Concatenate/1
  smoothingTimeCoMPos/1 -> MinimumJerkTrajectoryGenerator/2
  pos_vel_acc_jerk_CoM_des/1 -> "CoM6D ->  CoMXYZ5"/1

== system momentumBasedFlight/FLIGHT CONTROLLER (CORE) V2.5 - AERO/Flight State Machine/Compute Gains And References/Smooth CoM and Base References/Smooth Reference Orientations ==
  rot_vel_acc_jerk_base_des : Inport
  gainSmoothingBaseRot : Inport  Port=2
  Matrix Concatenate6 : Concatenate  NumInputs=4  Mode=Multidimensional array  ConcatenateDimension=2
  MinimumJerkTrajectoryGenerator : WBToolboxLibrary/Utilities/MinimumJerkTrajectoryGenerator  externalSettlingTime=off  settlingTime=Config.references.orientation.tSmoothingAngVel  sampleTime=Config.tStep  resetOnSettlingTime=off  firstDerivatives=on  secondDerivatives=on  explicitInitialValue=off
      settings: SourceProductName=WholeBodyToolbox
  Rotational PID Controller : Subsystem
  Selector : Selector  NumberOfDimensions=2  InputPortWidth=3  IndexOptions=Index vector (dialog),Index vector (dialog)  Indices=[1:3],[1:3]  OutputSizes=1,1
  rot_acc_vel_jerk_base_des_smooth : Outport  VectorParamsAs1DForOutWhenUnconnected=off
  wires:
  MinimumJerkTrajectoryGenerator/3 -> Matrix Concatenate6/4
  gainSmoothingBaseRot/1 -> Rotational PID Controller/2(gainSmoothingBaseRot)
  Selector/1 -> Rotational PID Controller/1(w_R_b_des)
  MinimumJerkTrajectoryGenerator/2 -> Matrix Concatenate6/3
  MinimumJerkTrajectoryGenerator/1 -> Matrix Concatenate6/2
  Rotational PID Controller/2(body_omega_b_des_smooth) -> MinimumJerkTrajectoryGenerator/1
  Rotational PID Controller/1(w_R_b_des_smooth) -> Matrix Concatenate6/1
  Matrix Concatenate6/1 -> rot_acc_vel_jerk_base_des_smooth/1
  rot_vel_acc_jerk_base_des/1 -> Selector/1

== system momentumBasedFlight/FLIGHT CONTROLLER (CORE) V2.5 - AERO/Flight State Machine/Compute Gains And References/Trajectory Generator/Overwrite turbo mode for high speed ==
  turbo_mode_gui : Inport
  turbo_mode_hs : Inport  Port=2
  Constant2 : Constant  Value=Config.high_speed_trajectory
  Switch : Switch  Criteria=u2 > Threshold
  turbo_mode : Outport
  wires:
  Switch/1 -> turbo_mode/1
  turbo_mode_gui/1 -> Switch/3
  turbo_mode_hs/1 -> Switch/1
  Constant2/1 -> Switch/2

== system momentumBasedFlight/FLIGHT CONTROLLER (CORE) V2.5 - AERO/Flight Controller RAL-HUMANOIDS V3.0 - AERODYNAMICS/Momentum Control for Flying/QP Solver and Integrate Contact Forces Derivative/Integrate the Contact Forces Derivative/deadZone ==
  u : Inport
  Constant : Constant  Value=Config.sat.deadZoneThreshold
  Deadzone Function : MATLAB Function  TreatAsAtomicUnit=on
  u_cut : Outport  VectorParamsAs1DForOutWhenUnconnected=off
  wires:
  Constant/1 -> Deadzone Function/2(thr)
  u/1 -> Deadzone Function/1(u)
  Deadzone Function/1(y) -> u_cut/1

== system momentumBasedFlight/FLIGHT CONTROLLER (CORE) V2.5 - AERO/Flight Controller RAL-HUMANOIDS V3.0 - AERODYNAMICS/Momentum Control for Flying/QP Solver and Integrate Contact Forces Derivative/QP momentumControl/QP momentumControl - balancing ==
  H : Inport
  g : Inport  Port=2
  ub : Inport  Port=3
  lb : Inport  Port=4
  Enable : EnablePort
  MatchSignalSizes : WBToolboxLibrary/Utilities/MatchSignalSizes
      settings: SourceProductName=WholeBodyToolbox
  QP : WBToolboxLibrary/Utilities/QP  lbA=off  ubA=off  lb=on  ub=on  computeObjVal=off  stopIfFails=off
      settings: SourceProductName=WholeBodyToolbox
  QPStatus_balancing : Outport  VectorParamsAs1DForOutWhenUnconnected=off
  QPOutput_balancing : Outport  Port=2  VectorParamsAs1DForOutWhenUnconnected=off
  wires:
  ub/1 -> QP/4
  g/1 -> QP/2, MatchSignalSizes/1
  H/1 -> QP/1
  QP/1 -> MatchSignalSizes/2
  MatchSignalSizes/1 -> QPOutput_balancing/1
  lb/1 -> QP/3
  QP/2 -> QPStatus_balancing/1

== system momentumBasedFlight/FLIGHT CONTROLLER (CORE) V2.5 - AERO/Flight Controller RAL-HUMANOIDS V3.0 - AERODYNAMICS/Momentum Control for Flying/QP Solver and Integrate Contact Forces Derivative/QP momentumControl/QP momentumControl - flight ==
  H : Inport
  g : Inport  Port=2
  ub : Inport  Port=3
  lb : Inport  Port=4
  Enable : EnablePort
  MatchSignalSizes : WBToolboxLibrary/Utilities/MatchSignalSizes
      settings: SourceProductName=WholeBodyToolbox
  QP : WBToolboxLibrary/Utilities/QP  lbA=off  ubA=off  lb=on  ub=on  computeObjVal=off  stopIfFails=off
      settings: SourceProductName=WholeBodyToolbox
  QPStatus_flight : Outport  VectorParamsAs1DForOutWhenUnconnected=off
  QPOutput_flight : Outport  Port=2  VectorParamsAs1DForOutWhenUnconnected=off
  wires:
  ub/1 -> QP/4
  g/1 -> QP/2, MatchSignalSizes/1
  H/1 -> QP/1
  QP/1 -> MatchSignalSizes/2
  MatchSignalSizes/1 -> QPOutput_flight/1
  lb/1 -> QP/3
  QP/2 -> QPStatus_flight/1

== system momentumBasedFlight/FLIGHT CONTROLLER (CORE) V2.5 - AERO/Flight Controller RAL-HUMANOIDS V3.0 - AERODYNAMICS/Momentum Control for Flying/QP Solver and Integrate Contact Forces Derivative/QP momentumControl/Select QP momentumControl Output ==
  QPStatus_balancing : Inport
  QPOutput_balancing : Inport  Port=2
  feetContactIsActive : Inport  Port=3
  QPStatus_flight : Inport  Port=4
  QPOutput_flight : Inport  Port=5
  Constant : Constant  Value=zeros(12,1)
  Demux : Demux  Outputs=[4;12;Config.N_DOF]
  Demux1 : Demux  Outputs=[4;Config.N_DOF]
  Switch{,1..3} (4 alike) : Switch  Criteria=u2 > Threshold
  jetsIntensitiesDot_star : Outport  VectorParamsAs1DForOutWhenUnconnected=off
  contactForcesDot_star : Outport  Port=2  VectorParamsAs1DForOutWhenUnconnected=off
  jointVel_star : Outport  Port=3  VectorParamsAs1DForOutWhenUnconnected=off
  exitFlagQP_momentumControl : Outport  Port=4  VectorParamsAs1DForOutWhenUnconnected=off
  wires:
  Demux1/2 -> Switch3/3
  Demux/3 -> Switch3/1
  Constant/1 -> Switch2/3
  Demux/2 -> Switch2/1
  Demux1/1 -> Switch1/3
  Demux/1 -> Switch1/1
  QPOutput_flight/1 -> Demux1/1
  QPOutput_balancing/1 -> Demux/1
  Switch/1 -> exitFlagQP_momentumControl/1
  QPStatus_flight/1 -> Switch/3
  QPStatus_balancing/1 -> Switch/1
  feetContactIsActive/1 -> Switch/2, Switch1/2, Switch2/2, Switch3/2
  Switch3/1 -> jointVel_star/1
  Switch1/1 -> jetsIntensitiesDot_star/1
  Switch2/1 -> contactForcesDot_star/1

== system momentumBasedFlight/FLIGHT CONTROLLER (CORE) V2.5 - AERO/Flight State Machine/Compute Gains And References/Smooth CoM and Base References/Smooth Reference Orientations/Rotational PID Controller ==
  w_R_b_des : Inport
  gainSmoothingBaseRot : Inport  Port=2
  Compute Rotation Matrix Derivative : MATLAB Function  TreatAsAtomicUnit=on
  Discrete-Time Integrator2 : DiscreteIntegrator  InitialConditionSource=external  InitialCondition=zeros(3,1)  SampleTime=Config.tStep  ICPrevOutput=DiscIntNeverNeededParam  ICPrevScaledInput=DiscIntNeverNeededParam
  "holder " : WBToolboxLibrary/Utilities/holder 
      settings: SourceProductName=WholeBodyToolbox
  w_R_b_des_smooth : Outport  VectorParamsAs1DForOutWhenUnconnected=off
  body_omega_b_des_smooth : Outport  Port=2  VectorParamsAs1DForOutWhenUnconnected=off
  wires:
  gainSmoothingBaseRot/1 -> Compute Rotation Matrix Derivative/1(gainSmoothingBaseRot)
  Compute Rotation Matrix Derivative/1(b_omega_b) -> body_omega_b_des_smooth/1
  w_R_b_des/1 -> Compute Rotation Matrix Derivative/2(w_R_b_des), "holder "/1
  Discrete-Time Integrator2/1 -> Compute Rotation Matrix Derivative/3(w_R_b), w_R_b_des_smooth/1
  Compute Rotation Matrix Derivative/2(RDot) -> Discrete-Time Integrator2/1
  "holder "/1 -> Discrete-Time Integrator2/2

== matlab function Visualizer/Task and Base Frame Kinematics/MATLAB Function1 ==
  data: RPY_Corr output double; rollPitchYaw input double
function RPY_Corr = correctYawAngleFCN(rollPitchYaw)

    RPY_Corr = correctYawAngle(rollPitchYaw);

end

== matlab function FLIGHT CONTROLLER (CORE) V2.5 - AERO/Flight State Machine/Compute Gains And References/Compute Gains/Diagonalize ==
  data: k input double; K output double
function K = diagonalMatrixFromVectorFCN(k)

    K = wbc.diagonalMatrixFromVector(k);
end

== matlab function Visualizer/Task and Base Frame Kinematics/MATLAB Function3 ==
  data: RPY_Corr output double; rollPitchYaw input double
function RPY_Corr = correctYawAngleFCN(rollPitchYaw)

    RPY_Corr = correctYawAngle(rollPitchYaw);

end

== matlab function Visualizer/Task and Base Frame Kinematics/Get RPY from rotation matrix  ==
  data: w_R_b input double; rollPitchYaw output double
function rollPitchYaw = rollPitchYawFromRotationFCN(w_R_b)

rollPitchYaw = wbc.rollPitchYawFromRotation(w_R_b);

end

== matlab function FLIGHT CONTROLLER (CORE) V2.5 - AERO/Flight State Machine/Compute Gains And References/Compute Gains/Diagonalize1 ==
  data: k input double; K output double
function K = diagonalMatrixFromVectorFCN(k)

    K = wbc.diagonalMatrixFromVector(k);
end

== matlab function Visualizer/Task and Base Frame Kinematics/Get RPY from rotation matrix ==
  data: w_R_b input double; rollPitchYaw output double
function rollPitchYaw = rollPitchYawFromRotationFCN(w_R_b)

rollPitchYaw = wbc.rollPitchYawFromRotation(w_R_b);

end

== matlab function Visualizer/Task and Base Frame Kinematics/Get RPY error norm ==
  data: rot_err input double; rotErr_norm output double
function rotErr_norm = normFCN(rot_err)

rotErr_norm = norm(rot_err);

end

== matlab function FLIGHT CONTROLLER (CORE) V2.5 - AERO/Flight State Machine/Compute Gains And References/Compute Gains/Diagonalize2 ==
  data: k input double; K output double
function K = diagonalMatrixFromVectorFCN(k)

    K = wbc.diagonalMatrixFromVector(k);
end

== matlab function FLIGHT CONTROLLER (CORE) V2.5 - AERO/Flight Controller RAL-HUMANOIDS V3.0 - AERODYNAMICS/Joint Torque Control for Flying/QP torqueControl/Process QP Inputs Torque Control ==
  data: HessianMatrixQP input double; H_balancing output double; gVectorQP input double; InequalityConstrMatrix input double; biasVectorInequalityConstr input double; g_balancing output double; ub_balancing output double; lb_balancing output double; Aeq_balancing output double; lbEq_balancing output double; ubEq_balancing output double; H_flight output double; g_flight output double; ub_flight output double; lb_flight output double; jointTorquesSaturation input double; Config parameter double
function [H_balancing,g_balancing,ub_balancing,lb_balancing,Aeq_balancing,lbEq_balancing,ubEq_balancing, ...
          H_flight,g_flight,ub_flight,lb_flight] = processQPinputTorqueControlFCN ...
                                                       (HessianMatrixQP,gVectorQP,InequalityConstrMatrix, ...
                                                        biasVectorInequalityConstr,jointTorquesSaturation,Config)   
   
[H_balancing,g_balancing,ub_balancing,lb_balancing,Aeq_balancing,lbEq_balancing,ubEq_balancing, ...
          H_flight,g_flight,ub_flight,lb_flight] = iRonCubLib.processQPinputTorqueControl ...
                                                       (HessianMatrixQP,gVectorQP,InequalityConstrMatrix, ...
                                                        biasVectorInequalityConstr,jointTorquesSaturation,Config);     
end

== matlab function Visualizer/Task and Base Frame Kinematics/MATLAB Function2 ==
  data: RPY_Corr output double; rollPitchYaw input double
function RPY_Corr = correctYawAngleFCN(rollPitchYaw)

    RPY_Corr = correctYawAngle(rollPitchYaw);

end

== matlab function FLIGHT CONTROLLER (CORE) V2.5 - AERO/Flight State Machine/Compute Gains And References/Compute Gains/Diagonalize3 ==
  data: k input double; K output double
function K = diagonalMatrixFromVectorFCN(k)

    K = wbc.diagonalMatrixFromVector(k);
end

== matlab function FLIGHT CONTROLLER (CORE) V2.5 - AERO/Flight State Machine/Compute Gains And References/Compute Gains/Diagonalize4 ==
  data: k input double; K output double
function K = diagonalMatrixFromVectorFCN(k)

    K = wbc.diagonalMatrixFromVector(k);
end

== matlab function FLIGHT CONTROLLER (CORE) V2.5 - AERO/Flight State Machine/Compute Gains And References/Trajectory Generator/Compute CoM and Base Rotation References ==
  data: posCoM_init input double; w_R_b_init input double; moveFront input double; pos_vel_acc_jerk_CoM_des output double; moveLateral input double; moveUpDown input double; rotateRoll input double; rotatePitch input double; rotateYaw input double; turbo_mode input double; goLandingPos input double; feetContactIsActive input double; oneFootIsInContact input double; t input double; Config parameter double; rot_vel_acc_jerk_base_des output double
function [pos_vel_acc_jerk_CoM_des, rot_vel_acc_jerk_base_des] = ...
             computeReferencesBaseAndCoMFCN(posCoM_init, w_R_b_init, moveFront, moveLateral, moveUpDown, rotateRoll, rotatePitch, ...
                                            rotateYaw, turbo_mode, goLandingPos, feetContactIsActive, oneFootIsInContact, t, Config)
                                     
    [pos_vel_acc_jerk_CoM_des, rot_vel_acc_jerk_base_des] = ...
        iRonCubLib.computeReferencesBaseAndCoM(posCoM_init, w_R_b_init, moveFront, moveLateral, moveUpDown, rotateRoll, rotatePitch, ...
                                               rotateYaw, turbo_mode, goLandingPos, feetContactIsActive, oneFootIsInContact, t, Config);
end

== matlab function FLIGHT CONTROLLER (CORE) V2.5 - AERO/Flight Controller RAL-HUMANOIDS V3.0 - AERODYNAMICS/Joint Torque Control for Flying/QP torqueControl/QP torqueControl - balancing/Combine Bounds and Inequalities ==
  data: AEq input double; AEq_combined output double; lbEq input double; ubEq input double; lb input double; ub input double; lbEq_combined output double; ubEq_combined output double
function [AEq_combined,lbEq_combined,ubEq_combined] = combineInputBoundsAndInequalitiesQPFCN(AEq,lbEq,ubEq,lb,ub)

   [AEq_combined,lbEq_combined,ubEq_combined] = iRonCubLib.combineInputBoundsAndInequalitiesQP(AEq,lbEq,ubEq,lb,ub);
end

== matlab function FLIGHT CONTROLLER (CORE) V2.5 - AERO/Flight Controller RAL-HUMANOIDS V3.0 - AERODYNAMICS/Joint Torque Control for Flying/Torque Derivative Saturation/Saturate Torque Derivative ==
  data: u input double; uSat output double; u_0 input double; tStep input double; uDotMax input double
function uSat = saturateInputDerivativeFCN(u, u_0, tStep, uDotMax)

    uSat = wbc.saturateInputDerivative(u, u_0, tStep, uDotMax);
end
